simulink model "Y_Model_20_Loads"  (R2018b)
settings: Solver=VariableStepAuto  StartTime=0.0  StopTime=sim_t  RelTol=1e-3
values from neighbouring files (symbols this model uses):
  dt = 5e-5    (= 5e-05)    [Y_multi_sim_loads.m]
  L = ones(num_sims, num_loads) * L_max    [Y_multi_sim_loads.m]
  P = rand(num_sims, num_loads) * (P_max - P_min) + P_min    [Y_multi_sim_loads.m]
  R = ones(num_sims, num_loads) * R_max    [Y_multi_sim_loads.m]
libraries: powerlib x270, powerlib_meascontrol x56
(part 2 of 4)

== system Y_Model_20_Loads/Load 34 ==
  Series RLC Branch3 : powerlib/Elements/Series RLC Branch  LConnTagsString=__new0  RConnTagsString=__new0  BranchType=RL  Resistance=R(4)  Inductance=L(4)  SetiL0=off  InitialCurrent=0  Capacitance=0  Setx0=off  InitialVoltage=0  Measurements=None
  Series RLC Branch4 : powerlib/Elements/Series RLC Branch  LConnTagsString=__new0  RConnTagsString=__new0  BranchType=RL  Resistance=R(4)  Inductance=L(4)  SetiL0=off  InitialCurrent=0  Capacitance=0  Setx0=off  InitialVoltage=0  Measurements=None
  Series RLC Branch5 : powerlib/Elements/Series RLC Branch  LConnTagsString=__new0  RConnTagsString=__new0  BranchType=RL  Resistance=R(4)  Inductance=L(4)  SetiL0=off  InitialCurrent=0  Capacitance=0  Setx0=off  InitialVoltage=0  Measurements=None
  Conn1 : PMIOPort  Side=Left
  Conn2 : PMIOPort  Port=2  Side=Right
  Conn3 : PMIOPort  Port=3  Side=Left
  Conn4 : PMIOPort  Port=4  Side=Right
  Conn5 : PMIOPort  Port=5  Side=Left
  Conn6 : PMIOPort  Port=6  Side=Right
  connections:
  Conn5/RConn1 -- Series RLC Branch5/LConn1
  Conn4/RConn1 -- Series RLC Branch4/RConn1
  Conn2/RConn1 -- Series RLC Branch3/RConn1
  Conn3/RConn1 -- Series RLC Branch4/LConn1
  Conn6/RConn1 -- Series RLC Branch5/RConn1
  Conn1/RConn1 -- Series RLC Branch3/LConn1

== system Y_Model_20_Loads/Load 35 ==
  Series RLC Branch3 : powerlib/Elements/Series RLC Branch  LConnTagsString=__new0  RConnTagsString=__new0  BranchType=RL  Resistance=R(1)  Inductance=L(1)  SetiL0=off  InitialCurrent=0  Capacitance=0  Setx0=off  InitialVoltage=0  Measurements=None
  Series RLC Branch4 : powerlib/Elements/Series RLC Branch  LConnTagsString=__new0  RConnTagsString=__new0  BranchType=RL  Resistance=R(1)  Inductance=L(1)  SetiL0=off  InitialCurrent=0  Capacitance=0  Setx0=off  InitialVoltage=0  Measurements=None
  Series RLC Branch5 : powerlib/Elements/Series RLC Branch  LConnTagsString=__new0  RConnTagsString=__new0  BranchType=RL  Resistance=R(1)  Inductance=L(1)  SetiL0=off  InitialCurrent=0  Capacitance=0  Setx0=off  InitialVoltage=0  Measurements=None
  Conn1 : PMIOPort  Side=Left
  Conn2 : PMIOPort  Port=2  Side=Right
  Conn3 : PMIOPort  Port=3  Side=Left
  Conn4 : PMIOPort  Port=4  Side=Right
  Conn5 : PMIOPort  Port=5  Side=Left
  Conn6 : PMIOPort  Port=6  Side=Right
  connections:
  Conn5/RConn1 -- Series RLC Branch5/LConn1
  Conn4/RConn1 -- Series RLC Branch4/RConn1
  Conn2/RConn1 -- Series RLC Branch3/RConn1
  Conn3/RConn1 -- Series RLC Branch4/LConn1
  Conn6/RConn1 -- Series RLC Branch5/RConn1
  Conn1/RConn1 -- Series RLC Branch3/LConn1

== system Y_Model_20_Loads/Load 36 ==
  Series RLC Branch3 : powerlib/Elements/Series RLC Branch  LConnTagsString=__new0  RConnTagsString=__new0  BranchType=RL  Resistance=R(3)  Inductance=L(3)  SetiL0=off  InitialCurrent=0  Capacitance=0  Setx0=off  InitialVoltage=0  Measurements=None
  Series RLC Branch4 : powerlib/Elements/Series RLC Branch  LConnTagsString=__new0  RConnTagsString=__new0  BranchType=RL  Resistance=R(3)  Inductance=L(3)  SetiL0=off  InitialCurrent=0  Capacitance=0  Setx0=off  InitialVoltage=0  Measurements=None
  Series RLC Branch5 : powerlib/Elements/Series RLC Branch  LConnTagsString=__new0  RConnTagsString=__new0  BranchType=RL  Resistance=R(3)  Inductance=L(3)  SetiL0=off  InitialCurrent=0  Capacitance=0  Setx0=off  InitialVoltage=0  Measurements=None
  Conn1 : PMIOPort  Side=Left
  Conn2 : PMIOPort  Port=2  Side=Right
  Conn3 : PMIOPort  Port=3  Side=Left
  Conn4 : PMIOPort  Port=4  Side=Right
  Conn5 : PMIOPort  Port=5  Side=Left
  Conn6 : PMIOPort  Port=6  Side=Right
  connections:
  Conn5/RConn1 -- Series RLC Branch5/LConn1
  Conn4/RConn1 -- Series RLC Branch4/RConn1
  Conn2/RConn1 -- Series RLC Branch3/RConn1
  Conn3/RConn1 -- Series RLC Branch4/LConn1
  Conn6/RConn1 -- Series RLC Branch5/RConn1
  Conn1/RConn1 -- Series RLC Branch3/LConn1

== system Y_Model_20_Loads/Load 37 ==
  Parallel RLC Load1 : powerlib/Elements/Parallel RLC Load  LConnTagsString=a  RConnTagsString=__new0  NominalVoltage=240  NominalFrequency=60  ActivePower=P(37)  InductivePower=P(37)/10  CapacitivePower=0  Setx0=off  InitialVoltage=0  SetiL0=off  InitialCurrent=0  Measurements=None  LoadType=constant Z
      settings: AttributesFormatString=\n  SourceProductName=Simscape Power Systems  SourceProductBaseCode=PS
  Parallel RLC Load2 : powerlib/Elements/Parallel RLC Load  LConnTagsString=a  RConnTagsString=__new0  NominalVoltage=240  NominalFrequency=60  ActivePower=P(37)  InductivePower=P(37)/10  CapacitivePower=0  Setx0=off  InitialVoltage=0  SetiL0=off  InitialCurrent=0  Measurements=None  LoadType=constant Z
      settings: AttributesFormatString=\n  SourceProductName=Simscape Power Systems  SourceProductBaseCode=PS
  Parallel RLC Load3 : powerlib/Elements/Parallel RLC Load  LConnTagsString=a  RConnTagsString=__new0  NominalVoltage=240  NominalFrequency=60  ActivePower=P(37)  InductivePower=P(37)/10  CapacitivePower=0  Setx0=off  InitialVoltage=0  SetiL0=off  InitialCurrent=0  Measurements=None  LoadType=constant Z
      settings: AttributesFormatString=\n  SourceProductName=Simscape Power Systems  SourceProductBaseCode=PS
  Conn1 : PMIOPort  Side=Left
  Conn2 : PMIOPort  Port=2  Side=Right
  Conn3 : PMIOPort  Port=3  Side=Left
  Conn4 : PMIOPort  Port=4  Side=Right
  Conn5 : PMIOPort  Port=5  Side=Left
  Conn6 : PMIOPort  Port=6  Side=Right
  connections:
  Parallel RLC Load1/RConn1 -- Conn4/RConn1
  Parallel RLC Load2/LConn1 -- Conn1/RConn1
  Parallel RLC Load2/RConn1 -- Conn2/RConn1
  Parallel RLC Load1/LConn1 -- Conn3/RConn1
  Parallel RLC Load3/LConn1 -- Conn5/RConn1
  Parallel RLC Load3/RConn1 -- Conn6/RConn1

== system Y_Model_20_Loads/Load 38 ==
  Series RLC Branch3 : powerlib/Elements/Series RLC Branch  LConnTagsString=__new0  RConnTagsString=__new0  BranchType=RL  Resistance=R(1)  Inductance=L(1)  SetiL0=off  InitialCurrent=0  Capacitance=0  Setx0=off  InitialVoltage=0  Measurements=None
  Series RLC Branch4 : powerlib/Elements/Series RLC Branch  LConnTagsString=__new0  RConnTagsString=__new0  BranchType=RL  Resistance=R(1)  Inductance=L(1)  SetiL0=off  InitialCurrent=0  Capacitance=0  Setx0=off  InitialVoltage=0  Measurements=None
  Series RLC Branch5 : powerlib/Elements/Series RLC Branch  LConnTagsString=__new0  RConnTagsString=__new0  BranchType=RL  Resistance=R(1)  Inductance=L(1)  SetiL0=off  InitialCurrent=0  Capacitance=0  Setx0=off  InitialVoltage=0  Measurements=None
  Conn1 : PMIOPort  Side=Left
  Conn2 : PMIOPort  Port=2  Side=Right
  Conn3 : PMIOPort  Port=3  Side=Left
  Conn4 : PMIOPort  Port=4  Side=Right
  Conn5 : PMIOPort  Port=5  Side=Left
  Conn6 : PMIOPort  Port=6  Side=Right
  connections:
  Conn5/RConn1 -- Series RLC Branch5/LConn1
  Conn4/RConn1 -- Series RLC Branch4/RConn1
  Conn2/RConn1 -- Series RLC Branch3/RConn1
  Conn3/RConn1 -- Series RLC Branch4/LConn1
  Conn6/RConn1 -- Series RLC Branch5/RConn1
  Conn1/RConn1 -- Series RLC Branch3/LConn1

== system Y_Model_20_Loads/Load 39 ==
  Series RLC Branch3 : powerlib/Elements/Series RLC Branch  LConnTagsString=__new0  RConnTagsString=__new0  BranchType=RL  Resistance=R(3)  Inductance=L(3)  SetiL0=off  InitialCurrent=0  Capacitance=0  Setx0=off  InitialVoltage=0  Measurements=None
  Series RLC Branch4 : powerlib/Elements/Series RLC Branch  LConnTagsString=__new0  RConnTagsString=__new0  BranchType=RL  Resistance=R(3)  Inductance=L(3)  SetiL0=off  InitialCurrent=0  Capacitance=0  Setx0=off  InitialVoltage=0  Measurements=None
  Series RLC Branch5 : powerlib/Elements/Series RLC Branch  LConnTagsString=__new0  RConnTagsString=__new0  BranchType=RL  Resistance=R(3)  Inductance=L(3)  SetiL0=off  InitialCurrent=0  Capacitance=0  Setx0=off  InitialVoltage=0  Measurements=None
  Conn1 : PMIOPort  Side=Left
  Conn2 : PMIOPort  Port=2  Side=Right
  Conn3 : PMIOPort  Port=3  Side=Left
  Conn4 : PMIOPort  Port=4  Side=Right
  Conn5 : PMIOPort  Port=5  Side=Left
  Conn6 : PMIOPort  Port=6  Side=Right
  connections:
  Conn5/RConn1 -- Series RLC Branch5/LConn1
  Conn4/RConn1 -- Series RLC Branch4/RConn1
  Conn2/RConn1 -- Series RLC Branch3/RConn1
  Conn3/RConn1 -- Series RLC Branch4/LConn1
  Conn6/RConn1 -- Series RLC Branch5/RConn1
  Conn1/RConn1 -- Series RLC Branch3/LConn1

== system Y_Model_20_Loads/Load 4 ==
  Series RLC Branch3 : powerlib/Elements/Series RLC Branch  LConnTagsString=__new0  RConnTagsString=__new0  BranchType=RL  Resistance=R(1)  Inductance=L(1)  SetiL0=off  InitialCurrent=0  Capacitance=0  Setx0=off  InitialVoltage=0  Measurements=None
  Series RLC Branch4 : powerlib/Elements/Series RLC Branch  LConnTagsString=__new0  RConnTagsString=__new0  BranchType=RL  Resistance=R(1)  Inductance=L(1)  SetiL0=off  InitialCurrent=0  Capacitance=0  Setx0=off  InitialVoltage=0  Measurements=None
  Series RLC Branch5 : powerlib/Elements/Series RLC Branch  LConnTagsString=__new0  RConnTagsString=__new0  BranchType=RL  Resistance=R(1)  Inductance=L(1)  SetiL0=off  InitialCurrent=0  Capacitance=0  Setx0=off  InitialVoltage=0  Measurements=None
  Conn1 : PMIOPort  Side=Left
  Conn2 : PMIOPort  Port=2  Side=Right
  Conn3 : PMIOPort  Port=3  Side=Left
  Conn4 : PMIOPort  Port=4  Side=Right
  Conn5 : PMIOPort  Port=5  Side=Left
  Conn6 : PMIOPort  Port=6  Side=Right
  connections:
  Conn5/RConn1 -- Series RLC Branch5/LConn1
  Conn4/RConn1 -- Series RLC Branch4/RConn1
  Conn2/RConn1 -- Series RLC Branch3/RConn1
  Conn3/RConn1 -- Series RLC Branch4/LConn1
  Conn6/RConn1 -- Series RLC Branch5/RConn1
  Conn1/RConn1 -- Series RLC Branch3/LConn1

== system Y_Model_20_Loads/Load 40 ==
  Parallel RLC Load1 : powerlib/Elements/Parallel RLC Load  LConnTagsString=a  RConnTagsString=__new0  NominalVoltage=240  NominalFrequency=60  ActivePower=P(40)  InductivePower=P(40)/10  CapacitivePower=0  Setx0=off  InitialVoltage=0  SetiL0=off  InitialCurrent=0  Measurements=None  LoadType=constant Z
      settings: AttributesFormatString=\n  SourceProductName=Simscape Power Systems  SourceProductBaseCode=PS
  Parallel RLC Load2 : powerlib/Elements/Parallel RLC Load  LConnTagsString=a  RConnTagsString=__new0  NominalVoltage=240  NominalFrequency=60  ActivePower=P(40)  InductivePower=P(40)/10  CapacitivePower=0  Setx0=off  InitialVoltage=0  SetiL0=off  InitialCurrent=0  Measurements=None  LoadType=constant Z
      settings: AttributesFormatString=\n  SourceProductName=Simscape Power Systems  SourceProductBaseCode=PS
  Parallel RLC Load3 : powerlib/Elements/Parallel RLC Load  LConnTagsString=a  RConnTagsString=__new0  NominalVoltage=240  NominalFrequency=60  ActivePower=P(40)  InductivePower=P(40)/10  CapacitivePower=0  Setx0=off  InitialVoltage=0  SetiL0=off  InitialCurrent=0  Measurements=None  LoadType=constant Z
      settings: AttributesFormatString=\n  SourceProductName=Simscape Power Systems  SourceProductBaseCode=PS
  Conn1 : PMIOPort  Side=Left
  Conn2 : PMIOPort  Port=2  Side=Right
  Conn3 : PMIOPort  Port=3  Side=Left
  Conn4 : PMIOPort  Port=4  Side=Right
  Conn5 : PMIOPort  Port=5  Side=Left
  Conn6 : PMIOPort  Port=6  Side=Right
  connections:
  Parallel RLC Load3/LConn1 -- Conn5/RConn1
  Parallel RLC Load1/RConn1 -- Conn4/RConn1
  Conn2/RConn1 -- Parallel RLC Load2/RConn1
  Parallel RLC Load1/LConn1 -- Conn3/RConn1
  Conn6/RConn1 -- Parallel RLC Load3/RConn1
  Parallel RLC Load2/LConn1 -- Conn1/RConn1

== system Y_Model_20_Loads/Load 42 ==
  Series RLC Branch3 : powerlib/Elements/Series RLC Branch  LConnTagsString=__new0  RConnTagsString=__new0  BranchType=RL  Resistance=R(3)  Inductance=L(3)  SetiL0=off  InitialCurrent=0  Capacitance=0  Setx0=off  InitialVoltage=0  Measurements=None
  Series RLC Branch4 : powerlib/Elements/Series RLC Branch  LConnTagsString=__new0  RConnTagsString=__new0  BranchType=RL  Resistance=R(3)  Inductance=L(3)  SetiL0=off  InitialCurrent=0  Capacitance=0  Setx0=off  InitialVoltage=0  Measurements=None
  Series RLC Branch5 : powerlib/Elements/Series RLC Branch  LConnTagsString=__new0  RConnTagsString=__new0  BranchType=RL  Resistance=R(3)  Inductance=L(3)  SetiL0=off  InitialCurrent=0  Capacitance=0  Setx0=off  InitialVoltage=0  Measurements=None
  Conn1 : PMIOPort  Side=Left
  Conn2 : PMIOPort  Port=2  Side=Right
  Conn3 : PMIOPort  Port=3  Side=Left
  Conn4 : PMIOPort  Port=4  Side=Right
  Conn5 : PMIOPort  Port=5  Side=Left
  Conn6 : PMIOPort  Port=6  Side=Right
  connections:
  Conn5/RConn1 -- Series RLC Branch5/LConn1
  Conn4/RConn1 -- Series RLC Branch4/RConn1
  Conn2/RConn1 -- Series RLC Branch3/RConn1
  Conn3/RConn1 -- Series RLC Branch4/LConn1
  Conn6/RConn1 -- Series RLC Branch5/RConn1
  Conn1/RConn1 -- Series RLC Branch3/LConn1

== system Y_Model_20_Loads/Load 43 ==
  Series RLC Branch3 : powerlib/Elements/Series RLC Branch  LConnTagsString=__new0  RConnTagsString=__new0  BranchType=RL  Resistance=R(4)  Inductance=L(4)  SetiL0=off  InitialCurrent=0  Capacitance=0  Setx0=off  InitialVoltage=0  Measurements=None
  Series RLC Branch4 : powerlib/Elements/Series RLC Branch  LConnTagsString=__new0  RConnTagsString=__new0  BranchType=RL  Resistance=R(4)  Inductance=L(4)  SetiL0=off  InitialCurrent=0  Capacitance=0  Setx0=off  InitialVoltage=0  Measurements=None
  Series RLC Branch5 : powerlib/Elements/Series RLC Branch  LConnTagsString=__new0  RConnTagsString=__new0  BranchType=RL  Resistance=R(4)  Inductance=L(4)  SetiL0=off  InitialCurrent=0  Capacitance=0  Setx0=off  InitialVoltage=0  Measurements=None
  Conn1 : PMIOPort  Side=Left
  Conn2 : PMIOPort  Port=2  Side=Right
  Conn3 : PMIOPort  Port=3  Side=Left
  Conn4 : PMIOPort  Port=4  Side=Right
  Conn5 : PMIOPort  Port=5  Side=Left
  Conn6 : PMIOPort  Port=6  Side=Right
  connections:
  Conn5/RConn1 -- Series RLC Branch5/LConn1
  Conn4/RConn1 -- Series RLC Branch4/RConn1
  Conn2/RConn1 -- Series RLC Branch3/RConn1
  Conn3/RConn1 -- Series RLC Branch4/LConn1
  Conn6/RConn1 -- Series RLC Branch5/RConn1
  Conn1/RConn1 -- Series RLC Branch3/LConn1

== system Y_Model_20_Loads/Load 44 ==
  Series RLC Branch3 : powerlib/Elements/Series RLC Branch  LConnTagsString=__new0  RConnTagsString=__new0  BranchType=RL  Resistance=R(1)  Inductance=L(1)  SetiL0=off  InitialCurrent=0  Capacitance=0  Setx0=off  InitialVoltage=0  Measurements=None
  Series RLC Branch4 : powerlib/Elements/Series RLC Branch  LConnTagsString=__new0  RConnTagsString=__new0  BranchType=RL  Resistance=R(1)  Inductance=L(1)  SetiL0=off  InitialCurrent=0  Capacitance=0  Setx0=off  InitialVoltage=0  Measurements=None
  Series RLC Branch5 : powerlib/Elements/Series RLC Branch  LConnTagsString=__new0  RConnTagsString=__new0  BranchType=RL  Resistance=R(1)  Inductance=L(1)  SetiL0=off  InitialCurrent=0  Capacitance=0  Setx0=off  InitialVoltage=0  Measurements=None
  Conn1 : PMIOPort  Side=Left
  Conn2 : PMIOPort  Port=2  Side=Right
  Conn3 : PMIOPort  Port=3  Side=Left
  Conn4 : PMIOPort  Port=4  Side=Right
  Conn5 : PMIOPort  Port=5  Side=Left
  Conn6 : PMIOPort  Port=6  Side=Right
  connections:
  Conn5/RConn1 -- Series RLC Branch5/LConn1
  Conn4/RConn1 -- Series RLC Branch4/RConn1
  Conn2/RConn1 -- Series RLC Branch3/RConn1
  Conn3/RConn1 -- Series RLC Branch4/LConn1
  Conn6/RConn1 -- Series RLC Branch5/RConn1
  Conn1/RConn1 -- Series RLC Branch3/LConn1

== system Y_Model_20_Loads/Load 45 ==
  Series RLC Branch3 : powerlib/Elements/Series RLC Branch  LConnTagsString=__new0  RConnTagsString=__new0  BranchType=RL  Resistance=R(3)  Inductance=L(3)  SetiL0=off  InitialCurrent=0  Capacitance=0  Setx0=off  InitialVoltage=0  Measurements=None
  Series RLC Branch4 : powerlib/Elements/Series RLC Branch  LConnTagsString=__new0  RConnTagsString=__new0  BranchType=RL  Resistance=R(3)  Inductance=L(3)  SetiL0=off  InitialCurrent=0  Capacitance=0  Setx0=off  InitialVoltage=0  Measurements=None
  Series RLC Branch5 : powerlib/Elements/Series RLC Branch  LConnTagsString=__new0  RConnTagsString=__new0  BranchType=RL  Resistance=R(3)  Inductance=L(3)  SetiL0=off  InitialCurrent=0  Capacitance=0  Setx0=off  InitialVoltage=0  Measurements=None
  Conn1 : PMIOPort  Side=Left
  Conn2 : PMIOPort  Port=2  Side=Right
  Conn3 : PMIOPort  Port=3  Side=Left
  Conn4 : PMIOPort  Port=4  Side=Right
  Conn5 : PMIOPort  Port=5  Side=Left
  Conn6 : PMIOPort  Port=6  Side=Right
  connections:
  Conn5/RConn1 -- Series RLC Branch5/LConn1
  Conn4/RConn1 -- Series RLC Branch4/RConn1
  Conn2/RConn1 -- Series RLC Branch3/RConn1
  Conn3/RConn1 -- Series RLC Branch4/LConn1
  Conn6/RConn1 -- Series RLC Branch5/RConn1
  Conn1/RConn1 -- Series RLC Branch3/LConn1

== system Y_Model_20_Loads/Load 46 ==
  Parallel RLC Load1 : powerlib/Elements/Parallel RLC Load  LConnTagsString=a  RConnTagsString=__new0  NominalVoltage=240  NominalFrequency=60  ActivePower=P(46)  InductivePower=P(46)/10  CapacitivePower=0  Setx0=off  InitialVoltage=0  SetiL0=off  InitialCurrent=0  Measurements=None  LoadType=constant Z
      settings: AttributesFormatString=\n  SourceProductName=Simscape Power Systems  SourceProductBaseCode=PS
  Parallel RLC Load2 : powerlib/Elements/Parallel RLC Load  LConnTagsString=a  RConnTagsString=__new0  NominalVoltage=240  NominalFrequency=60  ActivePower=P(46)  InductivePower=P(46)/10  CapacitivePower=0  Setx0=off  InitialVoltage=0  SetiL0=off  InitialCurrent=0  Measurements=None  LoadType=constant Z
      settings: AttributesFormatString=\n  SourceProductName=Simscape Power Systems  SourceProductBaseCode=PS
  Parallel RLC Load3 : powerlib/Elements/Parallel RLC Load  LConnTagsString=a  RConnTagsString=__new0  NominalVoltage=240  NominalFrequency=60  ActivePower=P(46)  InductivePower=P(46)/10  CapacitivePower=0  Setx0=off  InitialVoltage=0  SetiL0=off  InitialCurrent=0  Measurements=None  LoadType=constant Z
      settings: AttributesFormatString=\n  SourceProductName=Simscape Power Systems  SourceProductBaseCode=PS
  Conn1 : PMIOPort  Side=Left
  Conn2 : PMIOPort  Port=2  Side=Right
  Conn3 : PMIOPort  Port=3  Side=Left
  Conn4 : PMIOPort  Port=4  Side=Right
  Conn5 : PMIOPort  Port=5  Side=Left
  Conn6 : PMIOPort  Port=6  Side=Right
  connections:
  Conn1/RConn1 -- Parallel RLC Load1/LConn1
  Parallel RLC Load1/RConn1 -- Conn2/RConn1
  Parallel RLC Load2/LConn1 -- Conn3/RConn1
  Parallel RLC Load2/RConn1 -- Conn4/RConn1
  Parallel RLC Load3/LConn1 -- Conn5/RConn1
  Parallel RLC Load3/RConn1 -- Conn6/RConn1

== system Y_Model_20_Loads/Load 47 ==
  Series RLC Branch3 : powerlib/Elements/Series RLC Branch  LConnTagsString=__new0  RConnTagsString=__new0  BranchType=RL  Resistance=R(1)  Inductance=L(1)  SetiL0=off  InitialCurrent=0  Capacitance=0  Setx0=off  InitialVoltage=0  Measurements=None
  Series RLC Branch4 : powerlib/Elements/Series RLC Branch  LConnTagsString=__new0  RConnTagsString=__new0  BranchType=RL  Resistance=R(1)  Inductance=L(1)  SetiL0=off  InitialCurrent=0  Capacitance=0  Setx0=off  InitialVoltage=0  Measurements=None
  Series RLC Branch5 : powerlib/Elements/Series RLC Branch  LConnTagsString=__new0  RConnTagsString=__new0  BranchType=RL  Resistance=R(1)  Inductance=L(1)  SetiL0=off  InitialCurrent=0  Capacitance=0  Setx0=off  InitialVoltage=0  Measurements=None
  Conn1 : PMIOPort  Side=Left
  Conn2 : PMIOPort  Port=2  Side=Right
  Conn3 : PMIOPort  Port=3  Side=Left
  Conn4 : PMIOPort  Port=4  Side=Right
  Conn5 : PMIOPort  Port=5  Side=Left
  Conn6 : PMIOPort  Port=6  Side=Right
  connections:
  Conn5/RConn1 -- Series RLC Branch5/LConn1
  Conn4/RConn1 -- Series RLC Branch4/RConn1
  Conn2/RConn1 -- Series RLC Branch3/RConn1
  Conn3/RConn1 -- Series RLC Branch4/LConn1
  Conn6/RConn1 -- Series RLC Branch5/RConn1
  Conn1/RConn1 -- Series RLC Branch3/LConn1

== system Y_Model_20_Loads/Load 48 ==
  Series RLC Branch3 : powerlib/Elements/Series RLC Branch  LConnTagsString=__new0  RConnTagsString=__new0  BranchType=RL  Resistance=R(3)  Inductance=L(3)  SetiL0=off  InitialCurrent=0  Capacitance=0  Setx0=off  InitialVoltage=0  Measurements=None
  Series RLC Branch4 : powerlib/Elements/Series RLC Branch  LConnTagsString=__new0  RConnTagsString=__new0  BranchType=RL  Resistance=R(3)  Inductance=L(3)  SetiL0=off  InitialCurrent=0  Capacitance=0  Setx0=off  InitialVoltage=0  Measurements=None
  Series RLC Branch5 : powerlib/Elements/Series RLC Branch  LConnTagsString=__new0  RConnTagsString=__new0  BranchType=RL  Resistance=R(3)  Inductance=L(3)  SetiL0=off  InitialCurrent=0  Capacitance=0  Setx0=off  InitialVoltage=0  Measurements=None
  Conn1 : PMIOPort  Side=Left
  Conn2 : PMIOPort  Port=2  Side=Right
  Conn3 : PMIOPort  Port=3  Side=Left
  Conn4 : PMIOPort  Port=4  Side=Right
  Conn5 : PMIOPort  Port=5  Side=Left
  Conn6 : PMIOPort  Port=6  Side=Right
  connections:
  Conn5/RConn1 -- Series RLC Branch5/LConn1
  Conn4/RConn1 -- Series RLC Branch4/RConn1
  Conn2/RConn1 -- Series RLC Branch3/RConn1
  Conn3/RConn1 -- Series RLC Branch4/LConn1
  Conn6/RConn1 -- Series RLC Branch5/RConn1
  Conn1/RConn1 -- Series RLC Branch3/LConn1

== system Y_Model_20_Loads/Load 49 ==
  Parallel RLC Load1 : powerlib/Elements/Parallel RLC Load  LConnTagsString=a  RConnTagsString=__new0  NominalVoltage=240  NominalFrequency=60  ActivePower=P(49)  InductivePower=P(49)/10  CapacitivePower=0  Setx0=off  InitialVoltage=0  SetiL0=off  InitialCurrent=0  Measurements=None  LoadType=constant Z
      settings: AttributesFormatString=\n  SourceProductName=Simscape Power Systems  SourceProductBaseCode=PS
  Parallel RLC Load2 : powerlib/Elements/Parallel RLC Load  LConnTagsString=a  RConnTagsString=__new0  NominalVoltage=240  NominalFrequency=60  ActivePower=P(49)  InductivePower=P(49)/10  CapacitivePower=0  Setx0=off  InitialVoltage=0  SetiL0=off  InitialCurrent=0  Measurements=None  LoadType=constant Z
      settings: AttributesFormatString=\n  SourceProductName=Simscape Power Systems  SourceProductBaseCode=PS
  Parallel RLC Load3 : powerlib/Elements/Parallel RLC Load  LConnTagsString=a  RConnTagsString=__new0  NominalVoltage=240  NominalFrequency=60  ActivePower=P(49)  InductivePower=P(49)/10  CapacitivePower=0  Setx0=off  InitialVoltage=0  SetiL0=off  InitialCurrent=0  Measurements=None  LoadType=constant Z
      settings: AttributesFormatString=\n  SourceProductName=Simscape Power Systems  SourceProductBaseCode=PS
  Conn1 : PMIOPort  Side=Left
  Conn2 : PMIOPort  Port=2  Side=Right
  Conn3 : PMIOPort  Port=3  Side=Left
  Conn4 : PMIOPort  Port=4  Side=Right
  Conn5 : PMIOPort  Port=5  Side=Left
  Conn6 : PMIOPort  Port=6  Side=Right
  connections:
  Parallel RLC Load1/LConn1 -- Conn1/RConn1
  Parallel RLC Load1/RConn1 -- Conn2/RConn1
  Parallel RLC Load2/LConn1 -- Conn3/RConn1
  Parallel RLC Load2/RConn1 -- Conn4/RConn1
  Parallel RLC Load3/LConn1 -- Conn5/RConn1
  Parallel RLC Load3/RConn1 -- Conn6/RConn1

== system Y_Model_20_Loads/Load 5 ==
  Parallel RLC Load1 : powerlib/Elements/Parallel RLC Load  LConnTagsString=a  RConnTagsString=__new0  NominalVoltage=240  NominalFrequency=60  ActivePower=P(5)  InductivePower=P(5)/10  CapacitivePower=0  Setx0=off  InitialVoltage=0  SetiL0=off  InitialCurrent=0  Measurements=None  LoadType=constant Z
      settings: AttributesFormatString=\n  SourceProductName=Simscape Power Systems  SourceProductBaseCode=PS
  Parallel RLC Load2 : powerlib/Elements/Parallel RLC Load  LConnTagsString=a  RConnTagsString=__new0  NominalVoltage=240  NominalFrequency=60  ActivePower=P(5)  InductivePower=P(5)/10  CapacitivePower=0  Setx0=off  InitialVoltage=0  SetiL0=off  InitialCurrent=0  Measurements=None  LoadType=constant Z
      settings: AttributesFormatString=\n  SourceProductName=Simscape Power Systems  SourceProductBaseCode=PS
  Parallel RLC Load3 : powerlib/Elements/Parallel RLC Load  LConnTagsString=a  RConnTagsString=__new0  NominalVoltage=240  NominalFrequency=60  ActivePower=P(5)  InductivePower=P(5)/10  CapacitivePower=0  Setx0=off  InitialVoltage=0  SetiL0=off  InitialCurrent=0  Measurements=None  LoadType=constant Z
      settings: AttributesFormatString=\n  SourceProductName=Simscape Power Systems  SourceProductBaseCode=PS
  Conn1 : PMIOPort  Side=Left
  Conn2 : PMIOPort  Port=2  Side=Right
  Conn3 : PMIOPort  Port=3  Side=Left
  Conn4 : PMIOPort  Port=4  Side=Right
  Conn5 : PMIOPort  Port=5  Side=Left
  Conn6 : PMIOPort  Port=6  Side=Right
  connections:
  Parallel RLC Load2/LConn1 -- Conn5/RConn1
  Conn4/RConn1 -- Parallel RLC Load1/RConn1
  Parallel RLC Load3/RConn1 -- Conn2/RConn1
  Parallel RLC Load1/LConn1 -- Conn3/RConn1
  Conn6/RConn1 -- Parallel RLC Load2/RConn1
  Parallel RLC Load3/LConn1 -- Conn1/RConn1

== system Y_Model_20_Loads/Load 51 ==
  Series RLC Branch3 : powerlib/Elements/Series RLC Branch  LConnTagsString=__new0  RConnTagsString=__new0  BranchType=RL  Resistance=R(3)  Inductance=L(3)  SetiL0=off  InitialCurrent=0  Capacitance=0  Setx0=off  InitialVoltage=0  Measurements=None
  Series RLC Branch4 : powerlib/Elements/Series RLC Branch  LConnTagsString=__new0  RConnTagsString=__new0  BranchType=RL  Resistance=R(3)  Inductance=L(3)  SetiL0=off  InitialCurrent=0  Capacitance=0  Setx0=off  InitialVoltage=0  Measurements=None
  Series RLC Branch5 : powerlib/Elements/Series RLC Branch  LConnTagsString=__new0  RConnTagsString=__new0  BranchType=RL  Resistance=R(3)  Inductance=L(3)  SetiL0=off  InitialCurrent=0  Capacitance=0  Setx0=off  InitialVoltage=0  Measurements=None
  Conn1 : PMIOPort  Side=Left
  Conn2 : PMIOPort  Port=2  Side=Right
  Conn3 : PMIOPort  Port=3  Side=Left
  Conn4 : PMIOPort  Port=4  Side=Right
  Conn5 : PMIOPort  Port=5  Side=Left
  Conn6 : PMIOPort  Port=6  Side=Right
  connections:
  Conn5/RConn1 -- Series RLC Branch5/LConn1
  Conn4/RConn1 -- Series RLC Branch4/RConn1
  Conn2/RConn1 -- Series RLC Branch3/RConn1
  Conn3/RConn1 -- Series RLC Branch4/LConn1
  Conn6/RConn1 -- Series RLC Branch5/RConn1
  Conn1/RConn1 -- Series RLC Branch3/LConn1

== system Y_Model_20_Loads/Load 52 ==
  Series RLC Branch3 : powerlib/Elements/Series RLC Branch  LConnTagsString=__new0  RConnTagsString=__new0  BranchType=RL  Resistance=R(4)  Inductance=L(4)  SetiL0=off  InitialCurrent=0  Capacitance=0  Setx0=off  InitialVoltage=0  Measurements=None
  Series RLC Branch4 : powerlib/Elements/Series RLC Branch  LConnTagsString=__new0  RConnTagsString=__new0  BranchType=RL  Resistance=R(4)  Inductance=L(4)  SetiL0=off  InitialCurrent=0  Capacitance=0  Setx0=off  InitialVoltage=0  Measurements=None
  Series RLC Branch5 : powerlib/Elements/Series RLC Branch  LConnTagsString=__new0  RConnTagsString=__new0  BranchType=RL  Resistance=R(4)  Inductance=L(4)  SetiL0=off  InitialCurrent=0  Capacitance=0  Setx0=off  InitialVoltage=0  Measurements=None
  Conn1 : PMIOPort  Side=Left
  Conn2 : PMIOPort  Port=2  Side=Right
  Conn3 : PMIOPort  Port=3  Side=Left
  Conn4 : PMIOPort  Port=4  Side=Right
  Conn5 : PMIOPort  Port=5  Side=Left
  Conn6 : PMIOPort  Port=6  Side=Right
  connections:
  Conn5/RConn1 -- Series RLC Branch5/LConn1
  Conn4/RConn1 -- Series RLC Branch4/RConn1
  Conn2/RConn1 -- Series RLC Branch3/RConn1
  Conn3/RConn1 -- Series RLC Branch4/LConn1
  Conn6/RConn1 -- Series RLC Branch5/RConn1
  Conn1/RConn1 -- Series RLC Branch3/LConn1

== system Y_Model_20_Loads/Load 53 ==
  Series RLC Branch3 : powerlib/Elements/Series RLC Branch  LConnTagsString=__new0  RConnTagsString=__new0  BranchType=RL  Resistance=R(1)  Inductance=L(1)  SetiL0=off  InitialCurrent=0  Capacitance=0  Setx0=off  InitialVoltage=0  Measurements=None
  Series RLC Branch4 : powerlib/Elements/Series RLC Branch  LConnTagsString=__new0  RConnTagsString=__new0  BranchType=RL  Resistance=R(1)  Inductance=L(1)  SetiL0=off  InitialCurrent=0  Capacitance=0  Setx0=off  InitialVoltage=0  Measurements=None
  Series RLC Branch5 : powerlib/Elements/Series RLC Branch  LConnTagsString=__new0  RConnTagsString=__new0  BranchType=RL  Resistance=R(1)  Inductance=L(1)  SetiL0=off  InitialCurrent=0  Capacitance=0  Setx0=off  InitialVoltage=0  Measurements=None
  Conn1 : PMIOPort  Side=Left
  Conn2 : PMIOPort  Port=2  Side=Right
  Conn3 : PMIOPort  Port=3  Side=Left
  Conn4 : PMIOPort  Port=4  Side=Right
  Conn5 : PMIOPort  Port=5  Side=Left
  Conn6 : PMIOPort  Port=6  Side=Right
  connections:
  Conn5/RConn1 -- Series RLC Branch5/LConn1
  Conn4/RConn1 -- Series RLC Branch4/RConn1
  Conn2/RConn1 -- Series RLC Branch3/RConn1
  Conn3/RConn1 -- Series RLC Branch4/LConn1
  Conn6/RConn1 -- Series RLC Branch5/RConn1
  Conn1/RConn1 -- Series RLC Branch3/LConn1

== system Y_Model_20_Loads/Load 54 ==
  Series RLC Branch3 : powerlib/Elements/Series RLC Branch  LConnTagsString=__new0  RConnTagsString=__new0  BranchType=RL  Resistance=R(3)  Inductance=L(3)  SetiL0=off  InitialCurrent=0  Capacitance=0  Setx0=off  InitialVoltage=0  Measurements=None
  Series RLC Branch4 : powerlib/Elements/Series RLC Branch  LConnTagsString=__new0  RConnTagsString=__new0  BranchType=RL  Resistance=R(3)  Inductance=L(3)  SetiL0=off  InitialCurrent=0  Capacitance=0  Setx0=off  InitialVoltage=0  Measurements=None
  Series RLC Branch5 : powerlib/Elements/Series RLC Branch  LConnTagsString=__new0  RConnTagsString=__new0  BranchType=RL  Resistance=R(3)  Inductance=L(3)  SetiL0=off  InitialCurrent=0  Capacitance=0  Setx0=off  InitialVoltage=0  Measurements=None
  Conn1 : PMIOPort  Side=Left
  Conn2 : PMIOPort  Port=2  Side=Right
  Conn3 : PMIOPort  Port=3  Side=Left
  Conn4 : PMIOPort  Port=4  Side=Right
  Conn5 : PMIOPort  Port=5  Side=Left
  Conn6 : PMIOPort  Port=6  Side=Right
  connections:
  Conn5/RConn1 -- Series RLC Branch5/LConn1
  Conn4/RConn1 -- Series RLC Branch4/RConn1
  Conn2/RConn1 -- Series RLC Branch3/RConn1
  Conn3/RConn1 -- Series RLC Branch4/LConn1
  Conn6/RConn1 -- Series RLC Branch5/RConn1
  Conn1/RConn1 -- Series RLC Branch3/LConn1

== system Y_Model_20_Loads/Load 55 ==
  Parallel RLC Load1 : powerlib/Elements/Parallel RLC Load  LConnTagsString=a  RConnTagsString=__new0  NominalVoltage=240  NominalFrequency=60  ActivePower=P(55)  InductivePower=P(55)/10  CapacitivePower=0  Setx0=off  InitialVoltage=0  SetiL0=off  InitialCurrent=0  Measurements=None  LoadType=constant Z
      settings: AttributesFormatString=\n  SourceProductName=Simscape Power Systems  SourceProductBaseCode=PS
  Parallel RLC Load2 : powerlib/Elements/Parallel RLC Load  LConnTagsString=a  RConnTagsString=__new0  NominalVoltage=240  NominalFrequency=60  ActivePower=P(55)  InductivePower=P(55)/10  CapacitivePower=0  Setx0=off  InitialVoltage=0  SetiL0=off  InitialCurrent=0  Measurements=None  LoadType=constant Z
      settings: AttributesFormatString=\n  SourceProductName=Simscape Power Systems  SourceProductBaseCode=PS
  Parallel RLC Load3 : powerlib/Elements/Parallel RLC Load  LConnTagsString=a  RConnTagsString=__new0  NominalVoltage=240  NominalFrequency=60  ActivePower=P(55)  InductivePower=P(55)/10  CapacitivePower=0  Setx0=off  InitialVoltage=0  SetiL0=off  InitialCurrent=0  Measurements=None  LoadType=constant Z
      settings: AttributesFormatString=\n  SourceProductName=Simscape Power Systems  SourceProductBaseCode=PS
  Conn1 : PMIOPort  Side=Left
  Conn2 : PMIOPort  Port=2  Side=Right
  Conn3 : PMIOPort  Port=3  Side=Left
  Conn4 : PMIOPort  Port=4  Side=Right
  Conn5 : PMIOPort  Port=5  Side=Left
  Conn6 : PMIOPort  Port=6  Side=Right
  connections:
  Parallel RLC Load1/LConn1 -- Conn1/RConn1
  Parallel RLC Load1/RConn1 -- Conn2/RConn1
  Parallel RLC Load2/LConn1 -- Conn3/RConn1
  Parallel RLC Load2/RConn1 -- Conn4/RConn1
  Parallel RLC Load3/LConn1 -- Conn5/RConn1
  Parallel RLC Load3/RConn1 -- Conn6/RConn1

== system Y_Model_20_Loads/Load 56 ==
  Series RLC Branch3 : powerlib/Elements/Series RLC Branch  LConnTagsString=__new0  RConnTagsString=__new0  BranchType=RL  Resistance=R(1)  Inductance=L(1)  SetiL0=off  InitialCurrent=0  Capacitance=0  Setx0=off  InitialVoltage=0  Measurements=None
  Series RLC Branch4 : powerlib/Elements/Series RLC Branch  LConnTagsString=__new0  RConnTagsString=__new0  BranchType=RL  Resistance=R(1)  Inductance=L(1)  SetiL0=off  InitialCurrent=0  Capacitance=0  Setx0=off  InitialVoltage=0  Measurements=None
  Series RLC Branch5 : powerlib/Elements/Series RLC Branch  LConnTagsString=__new0  RConnTagsString=__new0  BranchType=RL  Resistance=R(1)  Inductance=L(1)  SetiL0=off  InitialCurrent=0  Capacitance=0  Setx0=off  InitialVoltage=0  Measurements=None
  Conn1 : PMIOPort  Side=Left
  Conn2 : PMIOPort  Port=2  Side=Right
  Conn3 : PMIOPort  Port=3  Side=Left
  Conn4 : PMIOPort  Port=4  Side=Right
  Conn5 : PMIOPort  Port=5  Side=Left
  Conn6 : PMIOPort  Port=6  Side=Right
  connections:
  Conn5/RConn1 -- Series RLC Branch5/LConn1
  Conn4/RConn1 -- Series RLC Branch4/RConn1
  Conn2/RConn1 -- Series RLC Branch3/RConn1
  Conn3/RConn1 -- Series RLC Branch4/LConn1
  Conn6/RConn1 -- Series RLC Branch5/RConn1
  Conn1/RConn1 -- Series RLC Branch3/LConn1

== system Y_Model_20_Loads/Load 57 ==
  Series RLC Branch3 : powerlib/Elements/Series RLC Branch  LConnTagsString=__new0  RConnTagsString=__new0  BranchType=RL  Resistance=R(3)  Inductance=L(3)  SetiL0=off  InitialCurrent=0  Capacitance=0  Setx0=off  InitialVoltage=0  Measurements=None
  Series RLC Branch4 : powerlib/Elements/Series RLC Branch  LConnTagsString=__new0  RConnTagsString=__new0  BranchType=RL  Resistance=R(3)  Inductance=L(3)  SetiL0=off  InitialCurrent=0  Capacitance=0  Setx0=off  InitialVoltage=0  Measurements=None
  Series RLC Branch5 : powerlib/Elements/Series RLC Branch  LConnTagsString=__new0  RConnTagsString=__new0  BranchType=RL  Resistance=R(3)  Inductance=L(3)  SetiL0=off  InitialCurrent=0  Capacitance=0  Setx0=off  InitialVoltage=0  Measurements=None
  Conn1 : PMIOPort  Side=Left
  Conn2 : PMIOPort  Port=2  Side=Right
  Conn3 : PMIOPort  Port=3  Side=Left
  Conn4 : PMIOPort  Port=4  Side=Right
  Conn5 : PMIOPort  Port=5  Side=Left
  Conn6 : PMIOPort  Port=6  Side=Right
  connections:
  Conn5/RConn1 -- Series RLC Branch5/LConn1
  Conn4/RConn1 -- Series RLC Branch4/RConn1
  Conn2/RConn1 -- Series RLC Branch3/RConn1
  Conn3/RConn1 -- Series RLC Branch4/LConn1
  Conn6/RConn1 -- Series RLC Branch5/RConn1
  Conn1/RConn1 -- Series RLC Branch3/LConn1

== system Y_Model_20_Loads/Load 58 ==
  Parallel RLC Load1 : powerlib/Elements/Parallel RLC Load  LConnTagsString=a  RConnTagsString=__new0  NominalVoltage=240  NominalFrequency=60  ActivePower=P(58)  InductivePower=P(58)/10  CapacitivePower=0  Setx0=off  InitialVoltage=0  SetiL0=off  InitialCurrent=0  Measurements=None  LoadType=constant Z
      settings: AttributesFormatString=\n  SourceProductName=Simscape Power Systems  SourceProductBaseCode=PS
  Parallel RLC Load2 : powerlib/Elements/Parallel RLC Load  LConnTagsString=a  RConnTagsString=__new0  NominalVoltage=240  NominalFrequency=60  ActivePower=P(58)  InductivePower=P(58)/10  CapacitivePower=0  Setx0=off  InitialVoltage=0  SetiL0=off  InitialCurrent=0  Measurements=None  LoadType=constant Z
      settings: AttributesFormatString=\n  SourceProductName=Simscape Power Systems  SourceProductBaseCode=PS
  Parallel RLC Load3 : powerlib/Elements/Parallel RLC Load  LConnTagsString=a  RConnTagsString=__new0  NominalVoltage=240  NominalFrequency=60  ActivePower=P(58)  InductivePower=P(58)/10  CapacitivePower=0  Setx0=off  InitialVoltage=0  SetiL0=off  InitialCurrent=0  Measurements=None  LoadType=constant Z
      settings: AttributesFormatString=\n  SourceProductName=Simscape Power Systems  SourceProductBaseCode=PS
  Conn1 : PMIOPort  Side=Left
  Conn2 : PMIOPort  Port=2  Side=Right
  Conn3 : PMIOPort  Port=3  Side=Left
  Conn4 : PMIOPort  Port=4  Side=Right
  Conn5 : PMIOPort  Port=5  Side=Left
  Conn6 : PMIOPort  Port=6  Side=Right
  connections:
  Parallel RLC Load3/LConn1 -- Conn5/RConn1
  Parallel RLC Load2/LConn1 -- Conn3/RConn1
  Parallel RLC Load1/LConn1 -- Conn1/RConn1
  Parallel RLC Load1/RConn1 -- Conn2/RConn1
  Parallel RLC Load2/RConn1 -- Conn4/RConn1
  Parallel RLC Load3/RConn1 -- Conn6/RConn1

== system Y_Model_20_Loads/Load 59 ==
  Series RLC Branch3 : powerlib/Elements/Series RLC Branch  LConnTagsString=__new0  RConnTagsString=__new0  BranchType=RL  Resistance=R(3)  Inductance=L(3)  SetiL0=off  InitialCurrent=0  Capacitance=0  Setx0=off  InitialVoltage=0  Measurements=None
  Series RLC Branch4 : powerlib/Elements/Series RLC Branch  LConnTagsString=__new0  RConnTagsString=__new0  BranchType=RL  Resistance=R(3)  Inductance=L(3)  SetiL0=off  InitialCurrent=0  Capacitance=0  Setx0=off  InitialVoltage=0  Measurements=None
  Series RLC Branch5 : powerlib/Elements/Series RLC Branch  LConnTagsString=__new0  RConnTagsString=__new0  BranchType=RL  Resistance=R(3)  Inductance=L(3)  SetiL0=off  InitialCurrent=0  Capacitance=0  Setx0=off  InitialVoltage=0  Measurements=None
  Conn1 : PMIOPort  Side=Left
  Conn2 : PMIOPort  Port=2  Side=Right
  Conn3 : PMIOPort  Port=3  Side=Left
  Conn4 : PMIOPort  Port=4  Side=Right
  Conn5 : PMIOPort  Port=5  Side=Left
  Conn6 : PMIOPort  Port=6  Side=Right
  connections:
  Conn5/RConn1 -- Series RLC Branch5/LConn1
  Conn4/RConn1 -- Series RLC Branch4/RConn1
  Conn2/RConn1 -- Series RLC Branch3/RConn1
  Conn3/RConn1 -- Series RLC Branch4/LConn1
  Conn6/RConn1 -- Series RLC Branch5/RConn1
  Conn1/RConn1 -- Series RLC Branch3/LConn1

== system Y_Model_20_Loads/Load 60 ==
  Series RLC Branch3 : powerlib/Elements/Series RLC Branch  LConnTagsString=__new0  RConnTagsString=__new0  BranchType=RL  Resistance=R(4)  Inductance=L(4)  SetiL0=off  InitialCurrent=0  Capacitance=0  Setx0=off  InitialVoltage=0  Measurements=None
  Series RLC Branch4 : powerlib/Elements/Series RLC Branch  LConnTagsString=__new0  RConnTagsString=__new0  BranchType=RL  Resistance=R(4)  Inductance=L(4)  SetiL0=off  InitialCurrent=0  Capacitance=0  Setx0=off  InitialVoltage=0  Measurements=None
  Series RLC Branch5 : powerlib/Elements/Series RLC Branch  LConnTagsString=__new0  RConnTagsString=__new0  BranchType=RL  Resistance=R(4)  Inductance=L(4)  SetiL0=off  InitialCurrent=0  Capacitance=0  Setx0=off  InitialVoltage=0  Measurements=None
  Conn1 : PMIOPort  Side=Left
  Conn2 : PMIOPort  Port=2  Side=Right
  Conn3 : PMIOPort  Port=3  Side=Left
  Conn4 : PMIOPort  Port=4  Side=Right
  Conn5 : PMIOPort  Port=5  Side=Left
  Conn6 : PMIOPort  Port=6  Side=Right
  connections:
  Conn5/RConn1 -- Series RLC Branch5/LConn1
  Conn4/RConn1 -- Series RLC Branch4/RConn1
  Conn2/RConn1 -- Series RLC Branch3/RConn1
  Conn3/RConn1 -- Series RLC Branch4/LConn1
  Conn6/RConn1 -- Series RLC Branch5/RConn1
  Conn1/RConn1 -- Series RLC Branch3/LConn1

== system Y_Model_20_Loads/Load 7 ==
  Series RLC Branch3 : powerlib/Elements/Series RLC Branch  LConnTagsString=__new0  RConnTagsString=__new0  BranchType=RL  Resistance=R(3)  Inductance=L(3)  SetiL0=off  InitialCurrent=0  Capacitance=0  Setx0=off  InitialVoltage=0  Measurements=None
  Series RLC Branch4 : powerlib/Elements/Series RLC Branch  LConnTagsString=__new0  RConnTagsString=__new0  BranchType=RL  Resistance=R(3)  Inductance=L(3)  SetiL0=off  InitialCurrent=0  Capacitance=0  Setx0=off  InitialVoltage=0  Measurements=None
  Series RLC Branch5 : powerlib/Elements/Series RLC Branch  LConnTagsString=__new0  RConnTagsString=__new0  BranchType=RL  Resistance=R(3)  Inductance=L(3)  SetiL0=off  InitialCurrent=0  Capacitance=0  Setx0=off  InitialVoltage=0  Measurements=None
  Conn1 : PMIOPort  Side=Left
  Conn2 : PMIOPort  Port=2  Side=Right
  Conn3 : PMIOPort  Port=3  Side=Left
  Conn4 : PMIOPort  Port=4  Side=Right
  Conn5 : PMIOPort  Port=5  Side=Left
  Conn6 : PMIOPort  Port=6  Side=Right
  connections:
  Conn5/RConn1 -- Series RLC Branch5/LConn1
  Conn4/RConn1 -- Series RLC Branch4/RConn1
  Conn2/RConn1 -- Series RLC Branch3/RConn1
  Conn3/RConn1 -- Series RLC Branch4/LConn1
  Conn6/RConn1 -- Series RLC Branch5/RConn1
  Conn1/RConn1 -- Series RLC Branch3/LConn1

== system Y_Model_20_Loads/Load 8 ==
  Series RLC Branch3 : powerlib/Elements/Series RLC Branch  LConnTagsString=__new0  RConnTagsString=__new0  BranchType=RL  Resistance=R(3)  Inductance=L(3)  SetiL0=off  InitialCurrent=0  Capacitance=0  Setx0=off  InitialVoltage=0  Measurements=None
  Series RLC Branch4 : powerlib/Elements/Series RLC Branch  LConnTagsString=__new0  RConnTagsString=__new0  BranchType=RL  Resistance=R(3)  Inductance=L(3)  SetiL0=off  InitialCurrent=0  Capacitance=0  Setx0=off  InitialVoltage=0  Measurements=None
  Series RLC Branch5 : powerlib/Elements/Series RLC Branch  LConnTagsString=__new0  RConnTagsString=__new0  BranchType=RL  Resistance=R(3)  Inductance=L(3)  SetiL0=off  InitialCurrent=0  Capacitance=0  Setx0=off  InitialVoltage=0  Measurements=None
  Conn1 : PMIOPort  Side=Left
  Conn2 : PMIOPort  Port=2  Side=Right
  Conn3 : PMIOPort  Port=3  Side=Left
  Conn4 : PMIOPort  Port=4  Side=Right
  Conn5 : PMIOPort  Port=5  Side=Left
  Conn6 : PMIOPort  Port=6  Side=Right
  connections:
  Conn5/RConn1 -- Series RLC Branch5/LConn1
  Conn4/RConn1 -- Series RLC Branch4/RConn1
  Conn2/RConn1 -- Series RLC Branch3/RConn1
  Conn3/RConn1 -- Series RLC Branch4/LConn1
  Conn6/RConn1 -- Series RLC Branch5/RConn1
  Conn1/RConn1 -- Series RLC Branch3/LConn1

== system Y_Model_20_Loads/Load 9 ==
  Series RLC Branch3 : powerlib/Elements/Series RLC Branch  LConnTagsString=__new0  RConnTagsString=__new0  BranchType=RL  Resistance=R(4)  Inductance=L(4)  SetiL0=off  InitialCurrent=0  Capacitance=0  Setx0=off  InitialVoltage=0  Measurements=None
  Series RLC Branch4 : powerlib/Elements/Series RLC Branch  LConnTagsString=__new0  RConnTagsString=__new0  BranchType=RL  Resistance=R(4)  Inductance=L(4)  SetiL0=off  InitialCurrent=0  Capacitance=0  Setx0=off  InitialVoltage=0  Measurements=None
  Series RLC Branch5 : powerlib/Elements/Series RLC Branch  LConnTagsString=__new0  RConnTagsString=__new0  BranchType=RL  Resistance=R(4)  Inductance=L(4)  SetiL0=off  InitialCurrent=0  Capacitance=0  Setx0=off  InitialVoltage=0  Measurements=None
  Conn1 : PMIOPort  Side=Left
  Conn2 : PMIOPort  Port=2  Side=Right
  Conn3 : PMIOPort  Port=3  Side=Left
  Conn4 : PMIOPort  Port=4  Side=Right
  Conn5 : PMIOPort  Port=5  Side=Left
  Conn6 : PMIOPort  Port=6  Side=Right
  connections:
  Conn5/RConn1 -- Series RLC Branch5/LConn1
  Conn4/RConn1 -- Series RLC Branch4/RConn1
  Conn2/RConn1 -- Series RLC Branch3/RConn1
  Conn3/RConn1 -- Series RLC Branch4/LConn1
  Conn6/RConn1 -- Series RLC Branch5/RConn1
  Conn1/RConn1 -- Series RLC Branch3/LConn1

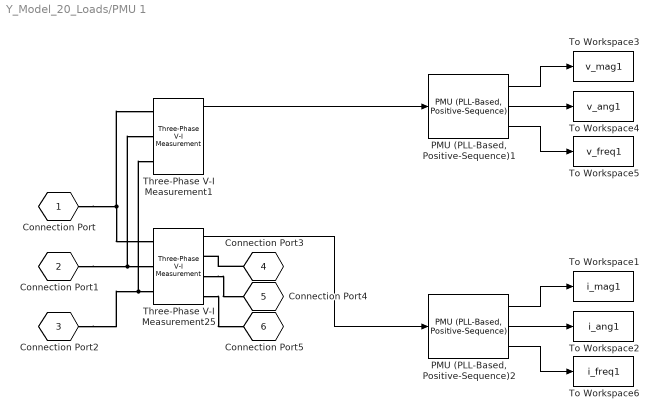
== system Y_Model_20_Loads/PMU 1 ==
  "PMU (PLL-Based, Positive-Sequence)1" : powerlib_meascontrol/Measurements/PMU (PLL-Based, Positive-Sequence)  nominalFrequency=50  samplingRate=64  reportingFactor=64
      settings: SourceProductName=Simscape Electrical  SourceProductBaseCode=PS
  "PMU (PLL-Based, Positive-Sequence)2" : powerlib_meascontrol/Measurements/PMU (PLL-Based, Positive-Sequence)  nominalFrequency=50  samplingRate=64  reportingFactor=64
      settings: SourceProductName=Simscape Electrical  SourceProductBaseCode=PS
  Three-Phase V-I Measurement1 : powerlib/Measurements/Three-Phase V-I Measurement  VoltageMeasurement=phase-to-ground  SetLabelV=off  LabelV=Vabc  Vpu=off  VpuLL=off  CurrentMeasurement=no  SetLabelI=off  LabelI=Iabc  Ipu=off  Pbase=100e6  Vbase=500e3  OutputType=Complex  PhasorSimulation=off  PSBequivalent=0
      settings: SourceProductName=Simscape Electrical
  Three-Phase V-I Measurement25 : powerlib/Measurements/Three-Phase V-I Measurement  VoltageMeasurement=no  SetLabelV=off  LabelV=Vabc  Vpu=off  VpuLL=off  CurrentMeasurement=yes  SetLabelI=off  LabelI=Iabc  Ipu=off  Pbase=100e6  Vbase=500e3  OutputType=Complex  PhasorSimulation=off  PSBequivalent=0
      settings: SourceProductName=Simscape Electrical
  To Workspace1 : ToWorkspace  VariableName=i_mag1  SampleTime=-1
  To Workspace2 : ToWorkspace  VariableName=i_ang1  SampleTime=-1
  To Workspace3 : ToWorkspace  VariableName=v_mag1  SampleTime=-1
  To Workspace4 : ToWorkspace  VariableName=v_ang1  SampleTime=-1
  To Workspace5 : ToWorkspace  VariableName=v_freq1  SampleTime=-1
  To Workspace6 : ToWorkspace  VariableName=i_freq1  SampleTime=-1
  Connection Port : PMIOPort  Tag=PMCPort  Side=Left
  Connection Port1 : PMIOPort  Tag=PMCPort  Port=2  Side=Left
  Connection Port2 : PMIOPort  Tag=PMCPort  Port=3  Side=Left
  Connection Port3 : PMIOPort  Tag=PMCPort  Port=4  Side=Right
  Connection Port4 : PMIOPort  Tag=PMCPort  Port=5  Side=Right
  Connection Port5 : PMIOPort  Tag=PMCPort  Port=6  Side=Right
  wires:
  "PMU (PLL-Based, Positive-Sequence)1"/3 -> To Workspace5/1
  "PMU (PLL-Based, Positive-Sequence)1"/2 -> To Workspace4/1
  "PMU (PLL-Based, Positive-Sequence)1"/1 -> To Workspace3/1
  "PMU (PLL-Based, Positive-Sequence)2"/3 -> To Workspace6/1
  "PMU (PLL-Based, Positive-Sequence)2"/1 -> To Workspace1/1
  "PMU (PLL-Based, Positive-Sequence)2"/2 -> To Workspace2/1
  Three-Phase V-I Measurement25/1 -> "PMU (PLL-Based, Positive-Sequence)2"/1
  Three-Phase V-I Measurement1/1 -> "PMU (PLL-Based, Positive-Sequence)1"/1
  connections:
  Connection Port/RConn1 -- Three-Phase V-I Measurement1/LConn1 -- Three-Phase V-I Measurement25/LConn1
  Connection Port1/RConn1 -- Three-Phase V-I Measurement25/LConn2 -- Three-Phase V-I Measurement1/LConn2
  Connection Port2/RConn1 -- Three-Phase V-I Measurement1/LConn3 -- Three-Phase V-I Measurement25/LConn3
  Connection Port3/RConn1 -- Three-Phase V-I Measurement25/RConn1
  Three-Phase V-I Measurement25/RConn2 -- Connection Port4/RConn1
  Three-Phase V-I Measurement25/RConn3 -- Connection Port5/RConn1

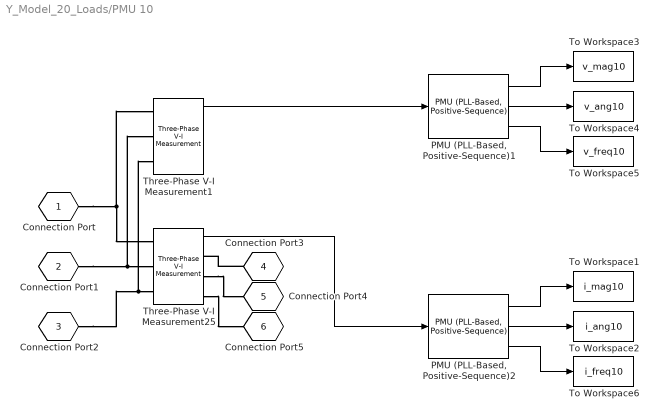
== system Y_Model_20_Loads/PMU 10 ==
  "PMU (PLL-Based, Positive-Sequence)1" : powerlib_meascontrol/Measurements/PMU (PLL-Based, Positive-Sequence)  nominalFrequency=50  samplingRate=64  reportingFactor=64
      settings: SourceProductName=Simscape Electrical  SourceProductBaseCode=PS
  "PMU (PLL-Based, Positive-Sequence)2" : powerlib_meascontrol/Measurements/PMU (PLL-Based, Positive-Sequence)  nominalFrequency=50  samplingRate=64  reportingFactor=64
      settings: SourceProductName=Simscape Electrical  SourceProductBaseCode=PS
  Three-Phase V-I Measurement1 : powerlib/Measurements/Three-Phase V-I Measurement  VoltageMeasurement=phase-to-ground  SetLabelV=off  LabelV=Vabc  Vpu=off  VpuLL=off  CurrentMeasurement=no  SetLabelI=off  LabelI=Iabc  Ipu=off  Pbase=100e6  Vbase=500e3  OutputType=Complex  PhasorSimulation=off  PSBequivalent=0
      settings: SourceProductName=Simscape Electrical
  Three-Phase V-I Measurement25 : powerlib/Measurements/Three-Phase V-I Measurement  VoltageMeasurement=no  SetLabelV=off  LabelV=Vabc  Vpu=off  VpuLL=off  CurrentMeasurement=yes  SetLabelI=off  LabelI=Iabc  Ipu=off  Pbase=100e6  Vbase=500e3  OutputType=Complex  PhasorSimulation=off  PSBequivalent=0
      settings: SourceProductName=Simscape Electrical
  To Workspace1 : ToWorkspace  VariableName=i_mag10  SampleTime=-1
  To Workspace2 : ToWorkspace  VariableName=i_ang10  SampleTime=-1
  To Workspace3 : ToWorkspace  VariableName=v_mag10  SampleTime=-1
  To Workspace4 : ToWorkspace  VariableName=v_ang10  SampleTime=-1
  To Workspace5 : ToWorkspace  VariableName=v_freq10  SampleTime=-1
  To Workspace6 : ToWorkspace  VariableName=i_freq10  SampleTime=-1
  Connection Port : PMIOPort  Tag=PMCPort  Side=Left
  Connection Port1 : PMIOPort  Tag=PMCPort  Port=2  Side=Left
  Connection Port2 : PMIOPort  Tag=PMCPort  Port=3  Side=Left
  Connection Port3 : PMIOPort  Tag=PMCPort  Port=4  Side=Right
  Connection Port4 : PMIOPort  Tag=PMCPort  Port=5  Side=Right
  Connection Port5 : PMIOPort  Tag=PMCPort  Port=6  Side=Right
  wires:
  "PMU (PLL-Based, Positive-Sequence)1"/3 -> To Workspace5/1
  "PMU (PLL-Based, Positive-Sequence)1"/2 -> To Workspace4/1
  "PMU (PLL-Based, Positive-Sequence)1"/1 -> To Workspace3/1
  "PMU (PLL-Based, Positive-Sequence)2"/3 -> To Workspace6/1
  "PMU (PLL-Based, Positive-Sequence)2"/1 -> To Workspace1/1
  "PMU (PLL-Based, Positive-Sequence)2"/2 -> To Workspace2/1
  Three-Phase V-I Measurement25/1 -> "PMU (PLL-Based, Positive-Sequence)2"/1
  Three-Phase V-I Measurement1/1 -> "PMU (PLL-Based, Positive-Sequence)1"/1
  connections:
  Three-Phase V-I Measurement25/LConn1 -- Connection Port/RConn1 -- Three-Phase V-I Measurement1/LConn1
  Connection Port1/RConn1 -- Three-Phase V-I Measurement1/LConn2 -- Three-Phase V-I Measurement25/LConn2
  Connection Port2/RConn1 -- Three-Phase V-I Measurement25/LConn3 -- Three-Phase V-I Measurement1/LConn3
  Connection Port3/RConn1 -- Three-Phase V-I Measurement25/RConn1
  Three-Phase V-I Measurement25/RConn2 -- Connection Port4/RConn1
  Three-Phase V-I Measurement25/RConn3 -- Connection Port5/RConn1
